simulink model "tia2_controller"  (R2023b)
settings: Solver=VariableStepAuto  StartTime=0.0  StopTime=5e-4  RelTol=1e-3
values from neighbouring files (symbols this model uses):
  fNoiseSampling = 1 / (rpFloor(2,1) - rpFloor(1,1))    [Laser_n_PID_initializer.m]
  fsampling = 125e6    (= 125000000)    [Laser_n_PID_initializer.m]
  s = estimate_iir_transfer_function(x,y,3,1)    [linearModelization.m]
libraries: slctrl_linear x3, spsFirstOrderFilterLib x2, cstblocks x1
settings Model: Creator=lastline  LastModifiedBy=lastline

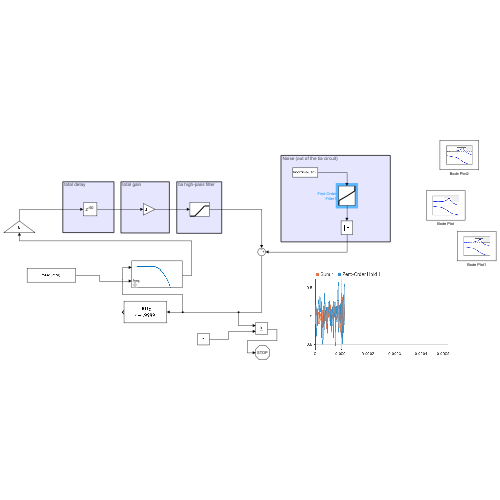
[thumbnail: Simulink's stored preview of the top-level diagram]
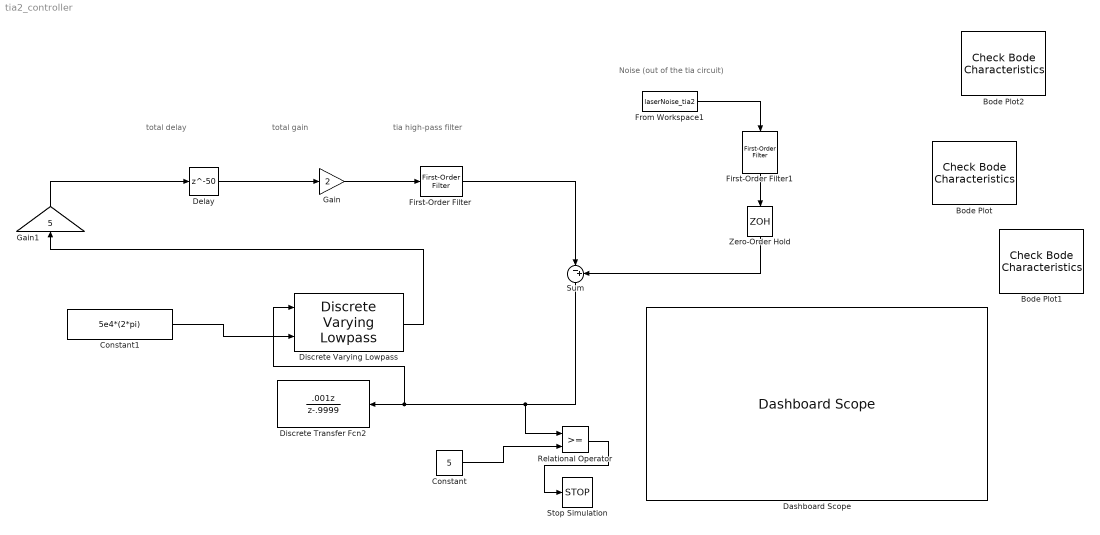
== system tia2_controller ==
  note: tia high-pass filter
  note: total gain
  note: total delay
  note: Noise (out of the tia circuit)
  Bode Plot : slctrl_linear/Check Bode  Characteristics  InstantiateOnLoad=on  SaveOperatingPoints=off  LinearizationIOs={'/Delay', 1, 'in', 'off', '';'/Gain1', 1, 'out', 'on', ''}  LinearizeAt=SnapshotTimes  SnapshotTimes=[0]  TriggerType=rising  SampleTime=auto  RateConversionMethod=zoh  PreWarpFreq=10  UseExactDelayModel=off  UseFullBlockNameLabels=off  UseBusSignalLabels=off  enabled=on  stopWhenAssertionFail=off  export=off  ViewDlgPos=[2001 546 510 390]  OpenViewOnLoad=on  LaunchViewOnOpen=on  FrequencyUnits=rad/s  MagnitudeUnits=dB  PhaseUnits=deg  TimeUnits=seconds  EnableUpperBound=off  UpperBoundFrequencies=[]  UpperBoundMagnitudes=[]  EnableLowerBound=off  LowerBoundFrequencies=[]  LowerBoundMagnitudes=[]
      settings: LibrarySourceBlock=slctrlblks/Linear Analysis Plots/Bode Plot  SaveToWorkspace=off  SaveName=sys
  Bode Plot1 : slctrl_linear/Check Bode  Characteristics  InstantiateOnLoad=on  SaveOperatingPoints=off  LinearizationIOs={'/Sum', 1, 'out', 'off', '';'/Delay', 1, 'in', 'off', ''}  LinearizeAt=SnapshotTimes  SnapshotTimes=[0]  TriggerType=rising  SampleTime=auto  RateConversionMethod=zoh  PreWarpFreq=10  UseExactDelayModel=off  UseFullBlockNameLabels=off  UseBusSignalLabels=off  enabled=on  stopWhenAssertionFail=off  export=off  ViewDlgPos=[2529 543 510 390]  OpenViewOnLoad=on  LaunchViewOnOpen=on  FrequencyUnits=rad/s  MagnitudeUnits=dB  PhaseUnits=deg  TimeUnits=seconds  EnableUpperBound=off  UpperBoundFrequencies=[]  UpperBoundMagnitudes=[]  EnableLowerBound=off  LowerBoundFrequencies=[]  LowerBoundMagnitudes=[]
      settings: LibrarySourceBlock=slctrlblks/Linear Analysis Plots/Bode Plot  SaveToWorkspace=off  SaveName=sys
  Bode Plot2 : slctrl_linear/Check Bode  Characteristics  InstantiateOnLoad=on  SaveOperatingPoints=off  LinearizationIOs={'/Sum', 1, 'in', 'off', '';'/Gain1', 1, 'out', 'on', ''}  LinearizeAt=SnapshotTimes  SnapshotTimes=[0]  TriggerType=rising  SampleTime=auto  RateConversionMethod=zoh  PreWarpFreq=10  UseExactDelayModel=off  UseFullBlockNameLabels=off  UseBusSignalLabels=off  enabled=on  stopWhenAssertionFail=off  export=off  ViewDlgPos=[2001 74 510 390]  OpenViewOnLoad=on  LaunchViewOnOpen=on  FrequencyUnits=rad/s  MagnitudeUnits=dB  PhaseUnits=deg  TimeUnits=seconds  EnableUpperBound=off  UpperBoundFrequencies=[]  UpperBoundMagnitudes=[]  EnableLowerBound=off  LowerBoundFrequencies=[]  LowerBoundMagnitudes=[]
      settings: LibrarySourceBlock=slctrlblks/Linear Analysis Plots/Bode Plot  SaveToWorkspace=off  SaveName=sys
  Constant : Constant  Value=5
  Constant1 : Constant  Value=5e4*(2*pi)
  Dashboard Scope : DashboardScope
  Delay : Delay  DelayLength=50  InitialCondition=0
  Discrete Transfer Fcn2 : DiscreteTransferFcn  Numerator=[.001 0]  Denominator=[1 -.9999]
  Discrete Varying Lowpass : cstblocks/Linear Parameter Varying/Discrete Varying Lowpass  N=1  w0=0  Ts=1/fsampling
  First-Order Filter : spsFirstOrderFilterLib/First-Order Filter  FilterType=Highpass  Tc=1e-3  Ts=0  Initialize=off  Vac_Init=[0, 0, 60]  Vdc_Init=0  PlotResponse=off  FreqRange="[0,  200,  1]"
  First-Order Filter1 : spsFirstOrderFilterLib/First-Order Filter  FilterType=Lowpass  Tc=1/(200e3)  Ts=0  Initialize=off  Vac_Init=[0, 0, 60]  Vdc_Init=0  PlotResponse=off  FreqRange="[0,  200,  1]"
  From Workspace1 : FromWorkspace  VariableName=laserNoise_tia2  SampleTime=1/fNoiseSampling  OutputAfterFinalValue=Setting to zero
  Gain : Gain  Gain=2
  Gain1 : Gain  Gain=5
  Relational Operator : RelationalOperator  OutDataTypeStr=boolean  RndMeth=Simplest  InputSameDT=off
  Stop Simulation : Stop
  Sum : Sum  Inputs=|-+
  Zero-Order Hold : ZeroOrderHold  SampleTime=1/fsampling
  wires:
  From Workspace1/1 -> First-Order Filter1/1
  First-Order Filter1/1 -> Zero-Order Hold/1
  First-Order Filter/1 -> Sum/1
  Gain/1 -> First-Order Filter/1
  Delay/1 -> Gain/1
  Sum/1 -> Relational Operator/1, Discrete Varying Lowpass/1, Discrete Transfer Fcn2/1
  Zero-Order Hold/1 -> Sum/2
  Relational Operator/1 -> Stop Simulation/1
  Constant/1 -> Relational Operator/2
  Constant1/1 -> Discrete Varying Lowpass/2
  Gain1/1 -> Delay/1
  Discrete Varying Lowpass/1 -> Gain1/1
